simulink model "pend_est_d"  (Simulink 5.0)
settings: Solver=ode45  StartTime=0.0  StopTime=10.0  RelTol=1e-3
values from neighbouring files (symbols this model uses):
  A = [-1 -2 0.5; 1 0 0; 0 1 0]    [ex_100.m]
undefined symbols (not defined in the file or in its folder): Ac, B, Bc, C, Cc, D, Dc, Ts
settings Model: Creator=kannan  LastModifiedBy=kannanm  ExtModeAutoUpdateStatusClock=off

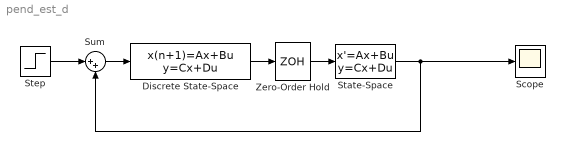
== system pend_est_d ==
  Discrete State-Space : DiscreteStateSpace  A=Ac  B=Bc  C=Cc  D=Dc  X0=[0 0 0 0]  SampleTime=Ts
  Scope : Scope
  State-Space : StateSpace  A=A  B=B  C=C  D=D  X0=[0 0.01 0 0]
  Step : Step  After=0  SampleTime=Ts
  Sum : Sum  Inputs=|++  SaturateOnIntegerOverflow=on
  Zero-Order Hold : ZeroOrderHold  SampleTime=Ts
  wires:
  Step/1 -> Sum/1
  State-Space/1 -> Scope/1, Sum/2
  Zero-Order Hold/1 -> State-Space/1
  Sum/1 -> Discrete State-Space/1
  Discrete State-Space/1 -> Zero-Order Hold/1
